simulink model "BallPlate"  (R2016a)
settings: Solver=FixedStepAuto  StartTime=0.0  StopTime=90  RelTol=1e-3
undefined symbols (not defined in the file): calib, DiscIntNeverNeededParam, TH_s, TH_v
libraries: simulink x17, ec_arm_cortex_a_lib x6, BallPlateLib x3, powerlib_meascontrol x1, dspnetwork x1
settings Model: SimulationMode=external  Creator=Arthur  LastModifiedBy=Arthur
settings SolverCC: PositivePriorityOrder=on
settings OptimizationCC: OptimizeModelRefInitCode=on  LifeSpan=1  MaxStackSize=64
settings HardwareCC: ProdBitPerPointer=32  ProdLargestAtomicInteger=Long  ProdLargestAtomicFloat=Double  ProdWordSize=32  ProdHWDeviceType=ARM Compatible->ARM Cortex
settings RTWCC: SystemTargetFile=ert.tlc  HardwareBoard=BeagleBone Black  TemplateMakefile=ert_default_tmf  GenerateReport=on  Toolchain=Linaro Toolchain v4.8  IncludeHyperlinkInReport=on  LaunchReport=on  GenerateTraceInfo=on  GenerateTraceReport=on  GenerateTraceReportSl=on  GenerateTraceReportSf=on  GenerateTraceReportEml=on
settings CodeAppCC: ForceParamTrailComments=on  IgnoreCustomStorageClasses=off  OperatorAnnotations=on  SimulinkDataObjDesc=on  SFDataObjDesc=on  MATLABFcnDesc=on  InsertBlockDesc=on  MATLABSourceComments=on
settings ERTTargetCC: SupportVariableSizeSignals=on  ExtMode=on  ExtModeMexArgs='192.168.7.2' 0 17725

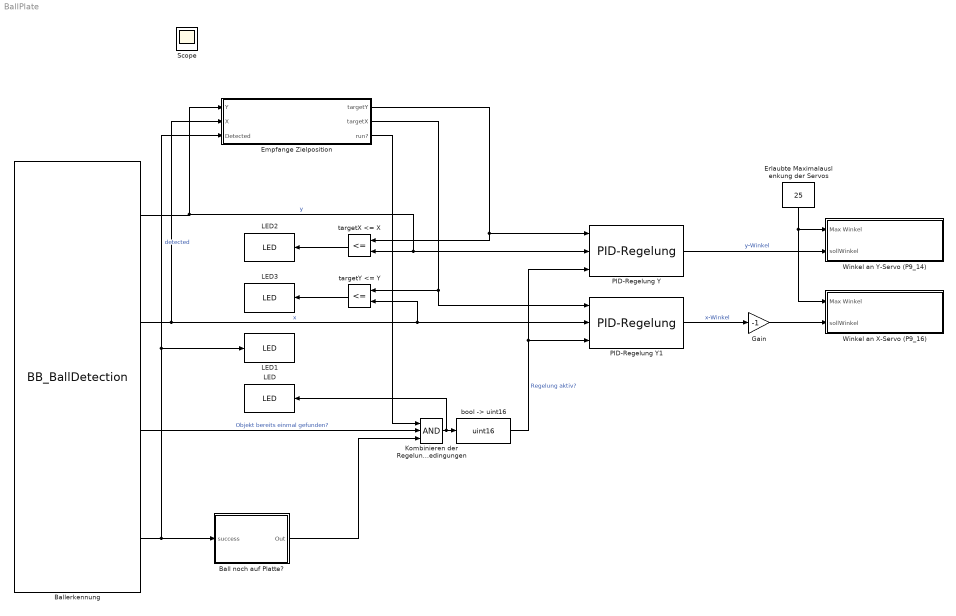
== system BallPlate ==
  Ball noch auf Platte? : Subsystem
  Ballerkennung : BallPlateLib/BB_BallDetection
  Empfange Zielposition : Subsystem
  Erlaubte Maximalauslenkung der Servos : Constant  Value=25
  Gain : Gain  Gain=-1
  Kombinieren der Regelungsbedingungen : Logic  Inputs=3  AllPortsSameDT=off  OutDataTypeStr=boolean
  LED : ec_arm_cortex_a_lib/LED  board=BeagleBone Black  led=USR0  blockPlatform=BeagleBone
  LED1 : ec_arm_cortex_a_lib/LED  board=BeagleBone Black  led=USR1  blockPlatform=BeagleBone
  LED2 : ec_arm_cortex_a_lib/LED  board=BeagleBone Black  led=USR2  blockPlatform=BeagleBone
  LED3 : ec_arm_cortex_a_lib/LED  board=BeagleBone Black  led=USR3  blockPlatform=BeagleBone
  PID-Regelung Y : BallPlateLib/PID-Regelung   p=46  i=20  d=9.2
  PID-Regelung Y1 : BallPlateLib/PID-Regelung   p=46  i=20  d=9.2
  Winkel an X-Servo (P9_16) : Subsystem
  Winkel an Y-Servo (P9_14) : Subsystem
  "bool -> uint16" : DataTypeConversion  OutDataTypeStr=uint16
  targetX <= X : RelationalOperator  Operator=<=  OutDataTypeStr=boolean
  targetY <= Y : RelationalOperator  Operator=<=  OutDataTypeStr=boolean
  Scope : Scope
  wires:
  Erlaubte Maximalauslenkung der Servos/1 -> Winkel an X-Servo (P9_16)/1(Max Winkel), Winkel an Y-Servo (P9_14)/1(Max Winkel)
  Ballerkennung/3 -> Kombinieren der Regelungsbedingungen/2  "Objekt bereits einmal gefunden?"
  Ballerkennung/1 -> Empfange Zielposition/1(Y), PID-Regelung Y/2, targetX <= X/2  "y"
  "bool -> uint16"/1 -> PID-Regelung Y1/3, PID-Regelung Y/3  "Regelung aktiv?"
  Ballerkennung/2 -> PID-Regelung Y1/2, targetY <= Y/2, Empfange Zielposition/2(X)  "x"
  PID-Regelung Y/1 -> Winkel an Y-Servo (P9_14)/2(sollWinkel)  "y-Winkel"
  Ballerkennung/4 -> Ball noch auf Platte?/1(success), Empfange Zielposition/3(Detected), LED1/1  "detected"
  Kombinieren der Regelungsbedingungen/1 -> LED/1, "bool -> uint16"/1
  PID-Regelung Y1/1 -> Gain/1  "x-Winkel"
  targetX <= X/1 -> LED2/1
  targetY <= Y/1 -> LED3/1
  Ball noch auf Platte?/1(Out) -> Kombinieren der Regelungsbedingungen/3
  Gain/1 -> Winkel an X-Servo (P9_16)/2(sollWinkel)
  Empfange Zielposition/1(targetY) -> targetX <= X/1, PID-Regelung Y/1
  Empfange Zielposition/2(targetX) -> PID-Regelung Y1/1, targetY <= Y/1
  Empfange Zielposition/3(run?) -> Kombinieren der Regelungsbedingungen/1

== system BallPlate/Ball noch auf Platte? ==
  success : Inport
  Stop condit. : simulink/Logic and Bit Operations/Compare To Constant  relop=<  const=0.33  OutDataTypeStr=boolean
  Zählung der Aufeinanderfolgenden Samples ohne erfolgreich Detection : DiscreteIntegrator  ExternalReset=falling  InitialConditionSetting=State (most efficient)  SampleTime=-1  ICPrevOutput=DiscIntNeverNeededParam  ICPrevScaledInput=DiscIntNeverNeededParam
  not : Logic  Operator=NOT  AllPortsSameDT=off  OutDataTypeStr=boolean
  to double : DataTypeConversion  OutDataTypeStr=double
  Out : Outport
  wires:
  success/1 -> not/1
  Stop condit./1 -> Out/1  "Ball noch auf Platte?"
  Zählung der Aufeinanderfolgenden Samples ohne erfolgreich Detection/1 -> Stop condit./1
  not/1 -> to double/1
  to double/1 -> Zählung der Aufeinanderfolgenden Samples ohne erfolgreich Detection/2, Zählung der Aufeinanderfolgenden Samples ohne erfolgreich Detection/1  "success"

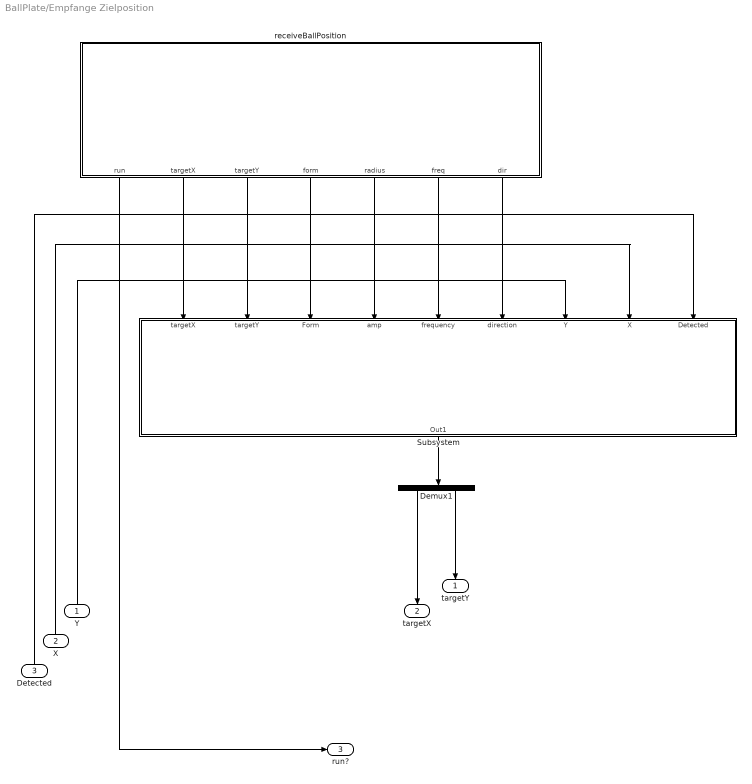
== system BallPlate/Empfange Zielposition ==
  Y : Inport
  X : Inport  Port=2
  Detected : Inport  Port=3
  Demux1 : Demux  Outputs=2
  Subsystem : Subsystem
  receiveBallPosition : Subsystem  AncestorBlock=BallPlateLib/receiveBallPosition
  targetY : Outport
  targetX : Outport  Port=2
  run? : Outport  Port=3
  wires:
  Demux1/1 -> targetX/1
  Demux1/2 -> targetY/1
  receiveBallPosition/1(run) -> run?/1
  receiveBallPosition/5(radius) -> Subsystem/4(amp)
  receiveBallPosition/3(targetY) -> Subsystem/2(targetY)
  receiveBallPosition/6(freq) -> Subsystem/5(frequency)
  receiveBallPosition/7(dir) -> Subsystem/6(direction)
  receiveBallPosition/2(targetX) -> Subsystem/1(targetX)
  receiveBallPosition/4(form) -> Subsystem/3(Form)
  Subsystem/1(Out1) -> Demux1/1
  Y/1 -> Subsystem/7(Y)
  X/1 -> Subsystem/8(X)
  Detected/1 -> Subsystem/9(Detected)

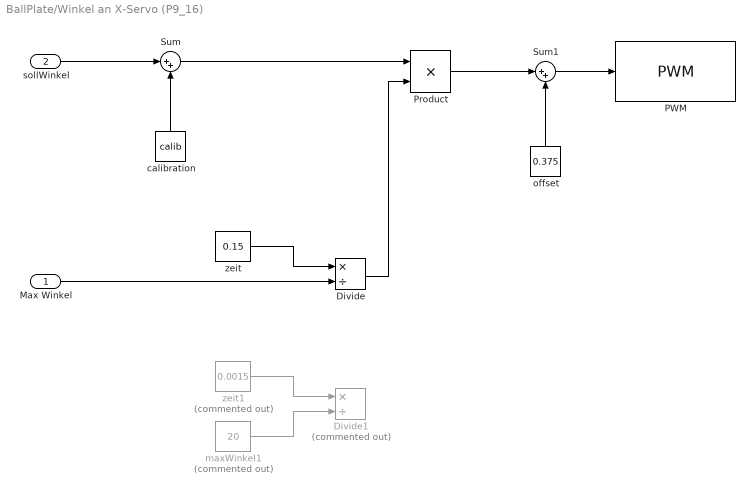
== system BallPlate/Winkel an X-Servo (P9_16) ==
  Max Winkel : Inport
  sollWinkel : Inport  Port=2
  Divide : Product  Inputs=*/
  Divide1 : Product  Commented=on  Inputs=*/
  PWM : ec_arm_cortex_a_lib/PWM  board=BeagleBone Black  pin=P9_16  frequency=250  polarity=Positive  blockPlatform=BeagleBone
  Product : Product
  Sum : Sum  Inputs=|++
  Sum1 : Sum  Inputs=|++
  calibration : Constant  Value=calib
  maxWinkel1 : Constant  Commented=on  Value=20
  offset : Constant  Value=0.375
  zeit : Constant  Value=0.15
  zeit1 : Constant  Commented=on  Value=0.0015
  wires:
  Sum/1 -> Product/1
  offset/1 -> Sum1/2
  calibration/1 -> Sum/2
  Product/1 -> Sum1/1
  sollWinkel/1 -> Sum/1
  Sum1/1 -> PWM/1
  zeit/1 -> Divide/1
  Max Winkel/1 -> Divide/2
  zeit1/1 -> Divide1/1
  maxWinkel1/1 -> Divide1/2
  Divide/1 -> Product/2

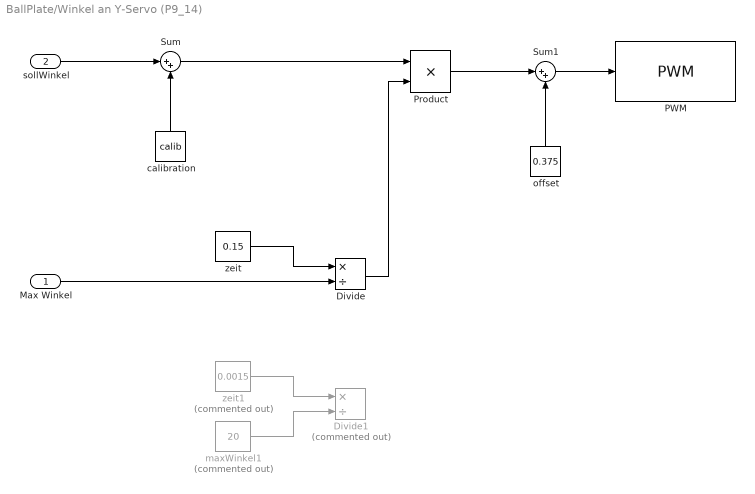
== system BallPlate/Winkel an Y-Servo (P9_14) ==
  Max Winkel : Inport
  sollWinkel : Inport  Port=2
  Divide : Product  Inputs=*/
  Divide1 : Product  Commented=on  Inputs=*/
  PWM : ec_arm_cortex_a_lib/PWM  board=BeagleBone Black  pin=P9_14  frequency=250  polarity=Positive  blockPlatform=BeagleBone
  Product : Product
  Sum : Sum  Inputs=|++
  Sum1 : Sum  Inputs=|++
  calibration : Constant  Value=calib
  maxWinkel1 : Constant  Commented=on  Value=20
  offset : Constant  Value=0.375
  zeit : Constant  Value=0.15
  zeit1 : Constant  Commented=on  Value=0.0015
  wires:
  Divide/1 -> Product/2
  maxWinkel1/1 -> Divide1/2
  zeit1/1 -> Divide1/1
  Max Winkel/1 -> Divide/2
  zeit/1 -> Divide/1
  Sum1/1 -> PWM/1
  sollWinkel/1 -> Sum/1
  Product/1 -> Sum1/1
  calibration/1 -> Sum/2
  offset/1 -> Sum1/2
  Sum/1 -> Product/1

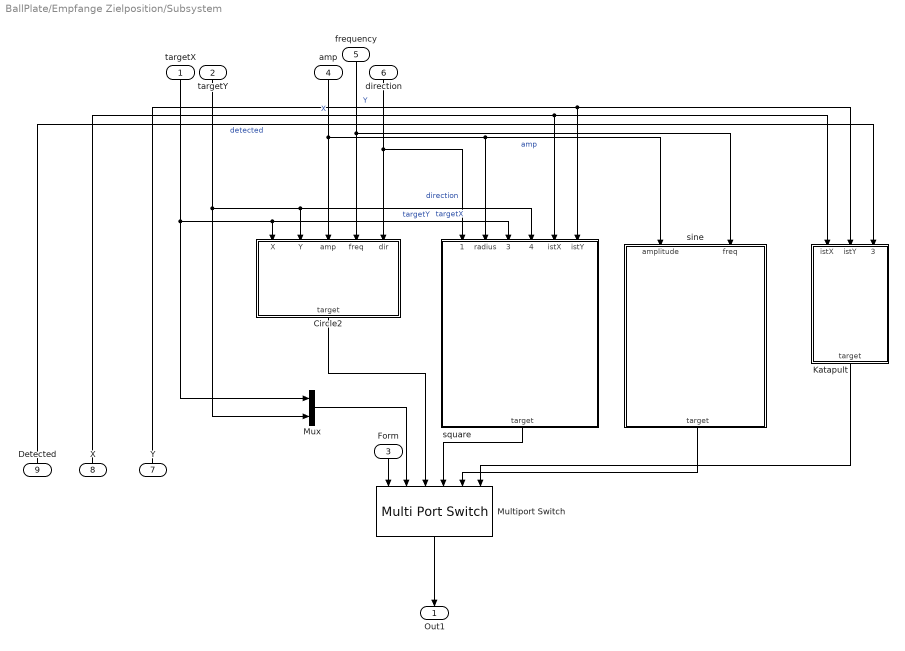
== system BallPlate/Empfange Zielposition/Subsystem ==
  targetX : Inport
  targetY : Inport  Port=2
  Form : Inport  Port=3
  amp : Inport  Port=4
  frequency : Inport  Port=5
  direction : Inport  Port=6
  Y : Inport  Port=7
  X : Inport  Port=8
  Detected : Inport  Port=9
  Circle2 : Subsystem
  Katapult : Subsystem
  Multiport Switch : MultiPortSwitch  Inputs=5
  Mux : Mux  Inputs=2
  sine : Subsystem
  square : Subsystem
  Out1 : Outport
  wires:
  Multiport Switch/1 -> Out1/1
  frequency/1 -> sine/2(freq), Circle2/4(freq)
  targetX/1 -> Mux/1, square/3(centerX), Circle2/1(X)  "targetX"
  Katapult/1(target) -> Multiport Switch/6
  direction/1 -> square/1(direction), Circle2/5(dir)  "direction"
  targetY/1 -> Mux/2, square/4(centerY), Circle2/2(Y)  "targetY"
  amp/1 -> sine/1(amplitude), square/2(radius), Circle2/3(amp)  "amp"
  X/1 -> Katapult/1(istX), square/5(istX)  "X"
  Y/1 -> Katapult/2(istY), square/6(istY)  "Y"
  Detected/1 -> Katapult/3(detected)  "detected"
  Form/1 -> Multiport Switch/1
  Mux/1 -> Multiport Switch/2
  square/1(target) -> Multiport Switch/4
  Circle2/1(target) -> Multiport Switch/3
  sine/1(target) -> Multiport Switch/5

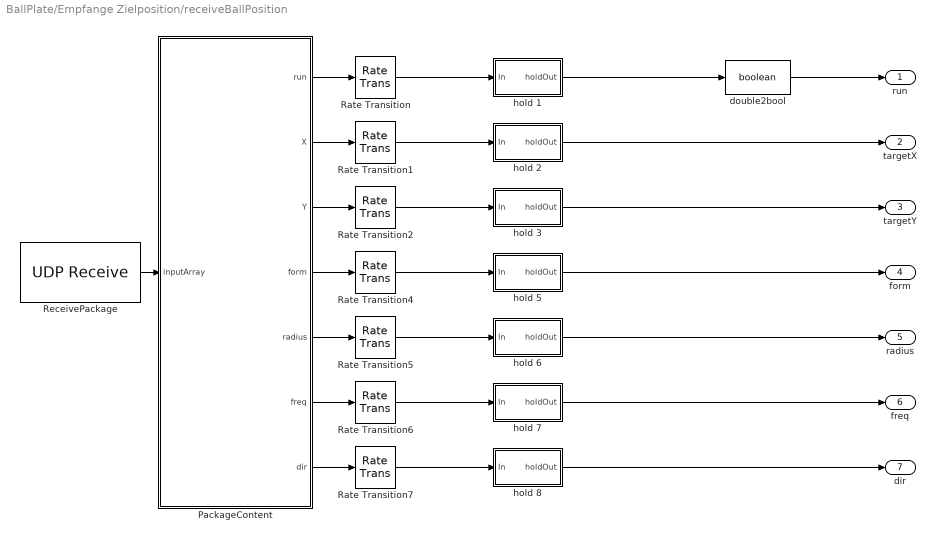
== system BallPlate/Empfange Zielposition/receiveBallPosition ==
  PackageContent : MATLAB Function  TreatAsAtomicUnit=on  SystemSampleTime=0.5
  Rate Transition{,1..2,4..7} (7 alike) : RateTransition  OutPortSampleTime=0.01
  ReceivePackage : dspnetwork/UDP Receive  localURL='0.0.0.0'  localPort=25000  remoteURL='0.0.0.0'  remotePort=-1  recvBufferSize=8192  dims=511  signalDatatype=double  isVarSize=on  showBlockingTime=on  blockingTime=0  sampletime=0.5  blockPlatform=BeagleBone
  double2bool : DataTypeConversion  OutDataTypeStr=boolean
  hold 1 : Subsystem
  hold 2 : Subsystem
  hold 3 : Subsystem
  hold 5 : Subsystem
  hold 6 : Subsystem
  hold 7 : Subsystem
  hold 8 : Subsystem
  run : Outport
  targetX : Outport  Port=2
  targetY : Outport  Port=3
  form : Outport  Port=4
  radius : Outport  Port=5
  freq : Outport  Port=6
  dir : Outport  Port=7
  wires:
  Rate Transition2/1 -> hold 3/1(In)
  Rate Transition1/1 -> hold 2/1(In)
  Rate Transition/1 -> hold 1/1(In)
  PackageContent/2(X) -> Rate Transition1/1
  ReceivePackage/1 -> PackageContent/1(inputArray)
  hold 2/1(holdOut) -> targetX/1
  hold 3/1(holdOut) -> targetY/1
  PackageContent/1(run) -> Rate Transition/1
  PackageContent/3(Y) -> Rate Transition2/1
  hold 1/1(holdOut) -> double2bool/1
  double2bool/1 -> run/1
  PackageContent/4(form) -> Rate Transition4/1
  Rate Transition4/1 -> hold 5/1(In)
  hold 5/1(holdOut) -> form/1
  PackageContent/5(radius) -> Rate Transition5/1
  Rate Transition5/1 -> hold 6/1(In)
  hold 6/1(holdOut) -> radius/1
  Rate Transition6/1 -> hold 7/1(In)
  hold 7/1(holdOut) -> freq/1
  Rate Transition7/1 -> hold 8/1(In)
  hold 8/1(holdOut) -> dir/1
  PackageContent/7(dir) -> Rate Transition7/1
  PackageContent/6(freq) -> Rate Transition6/1

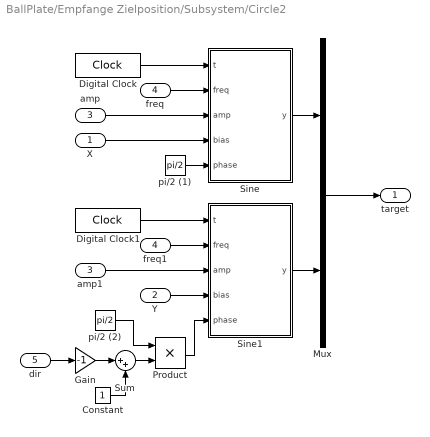
== system BallPlate/Empfange Zielposition/Subsystem/Circle2 ==
  X : Inport
  Y : Inport  Port=2
  amp : Inport  Port=3
  freq : Inport  Port=4
  dir : Inport  Port=5
  Constant : Constant
  Digital Clock : DigitalClock  SampleTime=0.01
  Digital Clock1 : DigitalClock  SampleTime=0.01
  Gain : Gain  Gain=-1
  Mux : Mux  Inputs=2
  Product : Product
  Sine : MATLAB Function  TreatAsAtomicUnit=on
  Sine1 : MATLAB Function  TreatAsAtomicUnit=on
  Sum : Sum  Inputs=|++
  amp1 : InportShadow  Port=3
  freq1 : InportShadow  Port=4
  pi/2 (1) : Constant  Value=pi/2
  pi/2 (2) : Constant  Value=pi/2
  target : Outport
  wires:
  Mux/1 -> target/1
  Digital Clock/1 -> Sine/1(t)
  Sine/1(y) -> Mux/1
  freq/1 -> Sine/2(freq)
  amp/1 -> Sine/3(amp)
  X/1 -> Sine/4(bias)
  Digital Clock1/1 -> Sine1/1(t)
  freq1/1 -> Sine1/2(freq)
  amp1/1 -> Sine1/3(amp)
  Sine1/1(y) -> Mux/2
  pi/2 (1)/1 -> Sine/5(phase)
  Product/1 -> Sine1/5(phase)
  pi/2 (2)/1 -> Product/1
  dir/1 -> Gain/1
  Constant/1 -> Sum/2
  Sum/1 -> Product/2
  Gain/1 -> Sum/1
  Y/1 -> Sine1/4(bias)

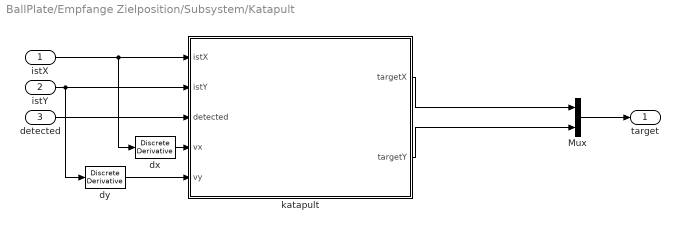
== system BallPlate/Empfange Zielposition/Subsystem/Katapult ==
  istX : Inport
  istY : Inport  Port=2
  detected : Inport  Port=3
  Mux : Mux  Inputs=2
  dx : simulink/Discrete/Discrete Derivative  gainval=1.0  ICPrevScaledInput=0.0  OutMin=[]  OutMax=[]  OutDataType=fixdt(1, 16)  OutScaling=2^-10  DoSatur=off
  dy : simulink/Discrete/Discrete Derivative  gainval=1.0  ICPrevScaledInput=0.0  OutMin=[]  OutMax=[]  OutDataType=fixdt(1, 16)  OutScaling=2^-10  DoSatur=off
  katapult : Stateflow chart  TreatAsAtomicUnit=on
  target : Outport
  wires:
  katapult/2(targetY) -> Mux/2
  katapult/1(targetX) -> Mux/1
  istY/1 -> katapult/2(istY), dy/1
  istX/1 -> dx/1, katapult/1(istX)
  detected/1 -> katapult/3(detected)
  Mux/1 -> target/1
  dx/1 -> katapult/4(vx)
  dy/1 -> katapult/5(vy)

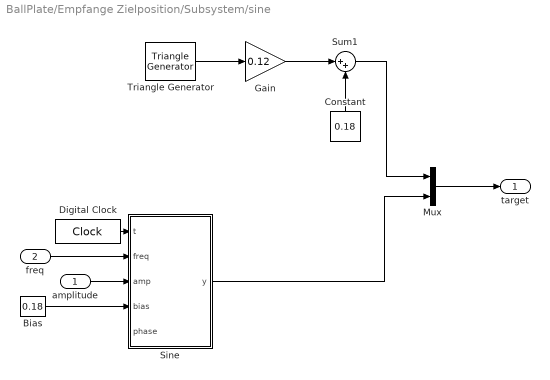
== system BallPlate/Empfange Zielposition/Subsystem/sine ==
  amplitude : Inport
  freq : Inport  Port=2
  Bias : Constant  Value=0.18
  Constant : Constant  Value=0.18
  Digital Clock : DigitalClock  SampleTime=0.01
  Gain : Gain  Gain=0.12
  Mux : Mux  Inputs=2
  Sine : MATLAB Function  TreatAsAtomicUnit=on
  Sum1 : Sum  Inputs=|++
  Triangle Generator : powerlib_meascontrol/Pulse & Signal Generators/Triangle Generator  Freq=0.4  Phase=0  Ts=0.01
  target : Outport
  wires:
  Mux/1 -> target/1
  Bias/1 -> Sine/4(bias)
  Sine/1(y) -> Mux/2
  amplitude/1 -> Sine/3(amp)
  Constant/1 -> Sum1/2
  Sum1/1 -> Mux/1
  Triangle Generator/1 -> Gain/1
  Gain/1 -> Sum1/1
  freq/1 -> Sine/2(freq)
  Digital Clock/1 -> Sine/1(t)

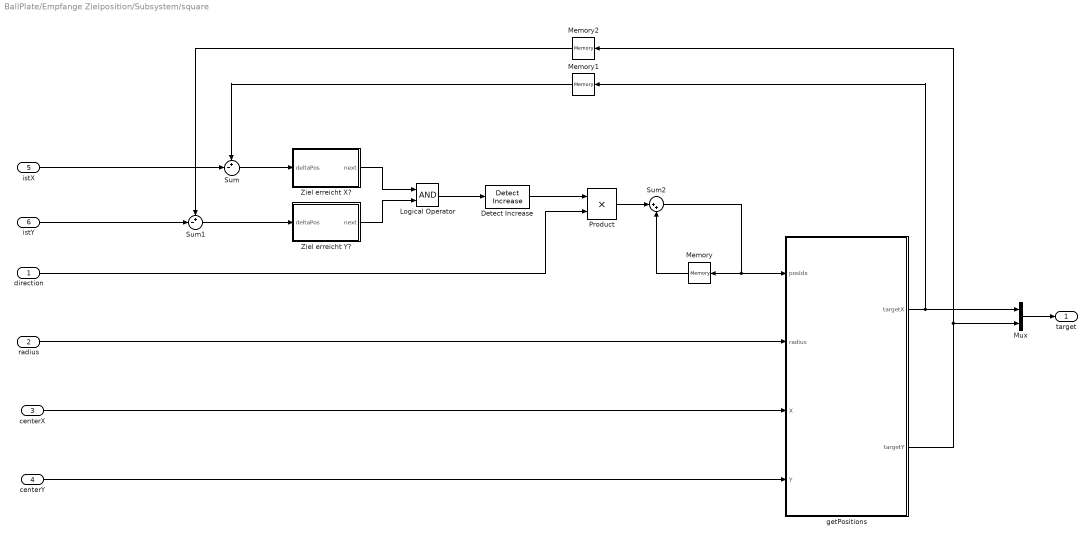
== system BallPlate/Empfange Zielposition/Subsystem/square ==
  direction : Inport
  radius : Inport  Port=2
  centerX : Inport  Port=3
  centerY : Inport  Port=4
  istX : Inport  Port=5
  istY : Inport  Port=6
  Detect Increase : simulink/Logic and Bit Operations/Detect Increase  vinit=0.0  OutDataTypeStr=boolean
  Logical Operator : Logic  AllPortsSameDT=off  OutDataTypeStr=boolean
  Memory : Memory  InheritSampleTime=on
  Memory1 : Memory  InheritSampleTime=on
  Memory2 : Memory  InheritSampleTime=on
  Mux : Mux  Inputs=2
  Product : Product
  Sum : Sum  Inputs=+-|
  Sum1 : Sum  Inputs=+-|
  Sum2 : Sum  Inputs=|++
  Ziel erreicht X? : Subsystem
  Ziel erreicht Y? : Subsystem
  getPositions : MATLAB Function  TreatAsAtomicUnit=on
  target : Outport
  wires:
  Mux/1 -> target/1
  radius/1 -> getPositions/2(radius)
  centerX/1 -> getPositions/3(X)
  centerY/1 -> getPositions/4(Y)
  getPositions/2(targetY) -> Memory2/1, Mux/2
  getPositions/1(targetX) -> Memory1/1, Mux/1
  Logical Operator/1 -> Detect Increase/1
  Ziel erreicht Y?/1(next) -> Logical Operator/2
  Sum1/1 -> Ziel erreicht Y?/1(deltaPos)
  direction/1 -> Product/2
  Ziel erreicht X?/1(next) -> Logical Operator/1
  Sum2/1 -> getPositions/1(posIdx), Memory/1
  Sum/1 -> Ziel erreicht X?/1(deltaPos)
  Detect Increase/1 -> Product/1
  Memory/1 -> Sum2/2
  istY/1 -> Sum1/2
  istX/1 -> Sum/2
  Product/1 -> Sum2/1
  Memory1/1 -> Sum/1
  Memory2/1 -> Sum1/1

== system BallPlate/Empfange Zielposition/receiveBallPosition/hold 1 ==
  In : Inport
  Memory : Memory
  Switch : Switch  Criteria=u2 ~= 0
  comp to -1 : simulink/Logic and Bit Operations/Compare To Constant  relop=~=  const=-1  OutDataTypeStr=boolean
  holdOut : Outport
  wires:
  Switch/1 -> holdOut/1, Memory/1
  Memory/1 -> Switch/3
  In/1 -> comp to -1/1, Switch/1
  comp to -1/1 -> Switch/2

== system BallPlate/Empfange Zielposition/receiveBallPosition/hold 2 ==
  In : Inport
  Memory : Memory
  Switch : Switch  Criteria=u2 ~= 0
  comp to -1 : simulink/Logic and Bit Operations/Compare To Constant  relop=~=  const=-1  OutDataTypeStr=boolean
  holdOut : Outport
  wires:
  comp to -1/1 -> Switch/2
  In/1 -> Switch/1, comp to -1/1
  Memory/1 -> Switch/3
  Switch/1 -> Memory/1, holdOut/1

== system BallPlate/Empfange Zielposition/receiveBallPosition/hold 3 ==
  In : Inport
  Memory : Memory
  Switch : Switch  Criteria=u2 ~= 0
  comp to -1 : simulink/Logic and Bit Operations/Compare To Constant  relop=~=  const=-1  OutDataTypeStr=boolean
  holdOut : Outport
  wires:
  Switch/1 -> holdOut/1, Memory/1
  Memory/1 -> Switch/3
  In/1 -> comp to -1/1, Switch/1
  comp to -1/1 -> Switch/2

== system BallPlate/Empfange Zielposition/receiveBallPosition/hold 5 ==
  In : Inport
  Memory : Memory
  Switch : Switch  Criteria=u2 ~= 0
  comp to -1 : simulink/Logic and Bit Operations/Compare To Constant  relop=~=  const=-1  OutDataTypeStr=boolean
  holdOut : Outport
  wires:
  Switch/1 -> holdOut/1, Memory/1
  Memory/1 -> Switch/3
  In/1 -> comp to -1/1, Switch/1
  comp to -1/1 -> Switch/2

== system BallPlate/Empfange Zielposition/receiveBallPosition/hold 6 ==
  In : Inport
  Memory : Memory
  Switch : Switch  Criteria=u2 ~= 0
  comp to -1 : simulink/Logic and Bit Operations/Compare To Constant  relop=~=  const=-1  OutDataTypeStr=boolean
  holdOut : Outport
  wires:
  comp to -1/1 -> Switch/2
  In/1 -> Switch/1, comp to -1/1
  Memory/1 -> Switch/3
  Switch/1 -> Memory/1, holdOut/1

== system BallPlate/Empfange Zielposition/receiveBallPosition/hold 7 ==
  In : Inport
  Memory : Memory
  Switch : Switch  Criteria=u2 ~= 0
  comp to -1 : simulink/Logic and Bit Operations/Compare To Constant  relop=~=  const=-1  OutDataTypeStr=boolean
  holdOut : Outport
  wires:
  Switch/1 -> holdOut/1, Memory/1
  Memory/1 -> Switch/3
  In/1 -> comp to -1/1, Switch/1
  comp to -1/1 -> Switch/2

== system BallPlate/Empfange Zielposition/receiveBallPosition/hold 8 ==
  In : Inport
  Memory : Memory
  Switch : Switch  Criteria=u2 ~= 0
  comp to -1 : simulink/Logic and Bit Operations/Compare To Constant  relop=~=  const=-2  OutDataTypeStr=boolean
  holdOut : Outport
  wires:
  comp to -1/1 -> Switch/2
  In/1 -> Switch/1, comp to -1/1
  Memory/1 -> Switch/3
  Switch/1 -> Memory/1, holdOut/1

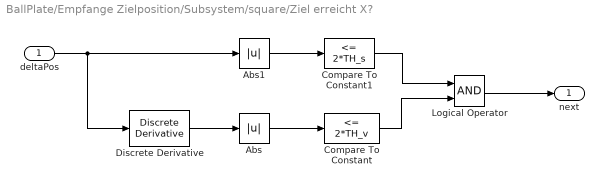
== system BallPlate/Empfange Zielposition/Subsystem/square/Ziel erreicht X? ==
  deltaPos : Inport
  Abs : Abs
  Abs1 : Abs
  Compare To Constant : simulink/Logic and Bit Operations/Compare To Constant  relop=<=  const=2*TH_v  OutDataTypeStr=boolean
  Compare To Constant1 : simulink/Logic and Bit Operations/Compare To Constant  relop=<=  const=2*TH_s  OutDataTypeStr=boolean
  Discrete Derivative : simulink/Discrete/Discrete Derivative  gainval=1.0  ICPrevScaledInput=0.0  OutMin=[]  OutMax=[]  OutDataType=fixdt(1, 16)  OutScaling=2^-10  DoSatur=off
  Logical Operator : Logic  AllPortsSameDT=off  OutDataTypeStr=boolean
  next : Outport
  wires:
  Abs1/1 -> Compare To Constant1/1
  Abs/1 -> Compare To Constant/1
  Logical Operator/1 -> next/1
  Compare To Constant1/1 -> Logical Operator/1
  Discrete Derivative/1 -> Abs/1
  deltaPos/1 -> Abs1/1, Discrete Derivative/1
  Compare To Constant/1 -> Logical Operator/2

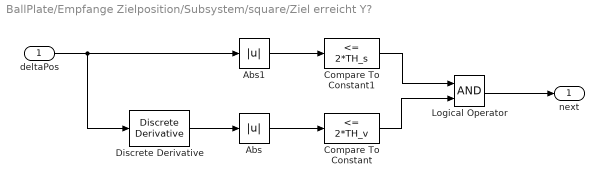
== system BallPlate/Empfange Zielposition/Subsystem/square/Ziel erreicht Y? ==
  deltaPos : Inport
  Abs : Abs
  Abs1 : Abs
  Compare To Constant : simulink/Logic and Bit Operations/Compare To Constant  relop=<=  const=2*TH_v  OutDataTypeStr=boolean
  Compare To Constant1 : simulink/Logic and Bit Operations/Compare To Constant  relop=<=  const=2*TH_s  OutDataTypeStr=boolean
  Discrete Derivative : simulink/Discrete/Discrete Derivative  gainval=1.0  ICPrevScaledInput=0.0  OutMin=[]  OutMax=[]  OutDataType=fixdt(1, 16)  OutScaling=2^-10  DoSatur=off
  Logical Operator : Logic  AllPortsSameDT=off  OutDataTypeStr=boolean
  next : Outport
  wires:
  Compare To Constant/1 -> Logical Operator/2
  deltaPos/1 -> Discrete Derivative/1, Abs1/1
  Discrete Derivative/1 -> Abs/1
  Compare To Constant1/1 -> Logical Operator/1
  Logical Operator/1 -> next/1
  Abs/1 -> Compare To Constant/1
  Abs1/1 -> Compare To Constant1/1

== matlab function BallPlate/Empfange Zielposition/Subsystem/Circle2/Sine ==
  data: t input; y output; freq input; amp input; bias input; phase input
function y = sine(t,freq,amp,bias,phase)

y = bias + amp * sin(freq*t + phase);

== matlab function BallPlate/Empfange Zielposition/Subsystem/square/getPositions ==
  data: posIdx input; targetX output; targetY output; radius input; X input; Y input
function [targetX,targetY] = fcn(posIdx, radius, X, Y)

posIdx = mod(posIdx,4);

targetX = -12.34;
targetY = 56.78;

switch posIdx
    
    case 0
        targetX = X - radius;
        targetY = Y - radius;    
    case 1
        targetX = X + radius;
        targetY = Y - radius;
    case 2
        targetX = X + radius;
        targetY = Y + radius;
    case 3
        targetX = X -radius;
        targetY = Y + radius;
end

== matlab function BallPlate/Empfange Zielposition/Subsystem/Circle2/Sine1 ==
  data: t input; y output; freq input; amp input; bias input; phase input
function y = sine(t,freq,amp,bias,phase)

y = bias + amp * sin(freq*t + phase);

== stateflow chart BallPlate/Empfange Zielposition/Subsystem/Katapult/katapult ==
  state iniTarget
    during:
    targetX = 0.25;
    targetY = 0.10;
  state throw
    during:
    targetX = 10;
    targetY = -10;
  state accelerate
    during:
    targetX =  -10;
    targetY = 10;
  (default) -> iniTarget
  (junction 16) -> iniTarget
  throw -> (junction 16) : [~detected]
  accelerate -> (junction 16) [order 2] : [~detected]
  iniTarget -> accelerate : [abs(targetX-istX) <= 0.02 && abs(targetY-istY) <= 0.02 && vx <= 0.1 && vy >= -0.1]
  accelerate -> throw [order 1] : [istX <= 0.13 && istY >= 0.2]
  data: istX input; istY input; targetX output; targetY output; detected input; vx input; vy input

== matlab function BallPlate/Empfange Zielposition/Subsystem/sine/Sine ==
  data: t input; y output; freq input; amp input; bias input; phase input
function y = sine(t,freq,amp,bias,phase)

y = bias + amp * sin(freq*t + phase);

== matlab function BallPlate/Empfange Zielposition/receiveBallPosition/PackageContent ==
  data: inputArray input [..255]; run output; X output; Y output; form output; radius output; freq output; dir output
function [run, X, Y, form, radius, freq, dir] = fcn(inputArray)

if ~isempty(inputArray)
    run = inputArray(1);
    X = inputArray(2);
    Y = inputArray(3);
    form = inputArray(4);
    radius = inputArray(5);
    freq = inputArray(6);
    dir = inputArray(7);
else
    run = -1;
    X = -1;
    Y = -1;
    form = -1;
    radius = -1;
    freq = -1;
    dir = -2;
end
